simulink model "connections"  (R2020a)
settings: Solver=FixedStepAuto  StartTime=0.0  StopTime=5000  FixedStep=0.1  RelTol=1e-3
values from neighbouring files (symbols this model uses):
  east_drift_limit = 2    [wave_parameters.mat]
  k_down = 1.3    [wave_parameters.mat]
  k_east = 2    [wave_parameters.mat]
  k_north = 2    [wave_parameters.mat]
  k_pitch = 3    [wave_parameters.mat]
  k_roll = 3    [wave_parameters.mat]
  k_yaw = 3    [wave_parameters.mat]
  north_drift_limit = 2    [wave_parameters.mat]
  numberOfBuses = 2    [init.m]
  numberOfGenerators = 4    [init.m]
  peak_frequency = 0.8    [wave_parameters.mat]
  wave_height = 1    [wave_parameters.mat]
  yaw_drift_limit = 0.174532925199    [wave_parameters.mat]
undefined symbols (not defined in the file or in its folder): east, magnitude, north, surge, sway, yaw
libraries: simulink x28, simulink_extras x18
(part 2 of 4)

== system connections/thruster_model/tunnel_thruster_3 ==
  desiredSetPoint : Inport  Unit=N
  desiredAzimuth : Inport  Port=2  Unit=deg
  Abs : Abs
  Add : Sum  Inputs=|+-
  Constant1 : Constant  Value=2
  Constant2 : Constant  Value=3
  Divide : Product
  Gain : Gain  Gain=144000
  Gain1 : Gain  Gain=1/100
  Gain2 : Gain  Gain=925000
  Integrator1 : Integrator
  Power : Math  Operator=pow  SignedPower=on  SaturateOnIntegerOverflow=on
  Power1 : Math  Operator=pow  SignedPower=on  SaturateOnIntegerOverflow=on
  Saturation : Saturate  UpperLimit=100  LowerLimit=-100
  Sign : Signum
  p : Outport  Unit=W  VectorParamsAs1DForOutWhenUnconnected=off  BusOutputAsStruct=on
  thrust : Outport  Port=2  Unit=N  VectorParamsAs1DForOutWhenUnconnected=off
  azimuth : Outport  Port=3  Unit=deg  VectorParamsAs1DForOutWhenUnconnected=off  BusOutputAsStruct=on
  sensorFeedback : Outport  Port=4  Unit=deg  VectorParamsAs1DForOutWhenUnconnected=off  BusOutputAsStruct=on
  wires:
  Abs/1 -> p/1
  Constant1/1 -> Power/2  "q"
  Sign/1 -> Divide/1
  Constant2/1 -> Power1/2  "q"
  Gain2/1 -> Abs/1  "power"
  Gain/1 -> Divide/2  "thrust"
  Power/1 -> Gain/1
  desiredSetPoint/1 -> Saturation/1  "thrustSetPoint"
  Power1/1 -> Gain2/1
  Divide/1 -> thrust/1
  Saturation/1 -> Gain1/1
  Integrator1/1 -> Add/2, Sign/1, sensorFeedback/1, Power1/1, Power/1
  Add/1 -> Integrator1/1
  Gain1/1 -> Add/1
  desiredAzimuth/1 -> azimuth/1

== system connections/vessel_model/VesselDynamics ==
  ExternalForceAndMoments : Inport
  6DOFRotationMatrix : Subsystem
  Add : Sum  Inputs=+--
  Demux : Demux  Outputs=3
  MatrixMultiply : Product  Inputs=/*  Multiplication=Matrix(*)
  MatrixMultiply2 : Product  Inputs=**  Multiplication=Matrix(*)
  Scope : Scope
  Selector : Selector  NumberOfDimensions=2  InputPortWidth=3  IndexOptions=Select all,Index vector (dialog)  Indices=[1 3],1  OutputSizes=1,1
  Selector1 : Selector  InputPortWidth=6  IndexOptions=Index vector (dialog)  Indices=[4 5 6]  OutputSizes=1
  Vessel mass matrix : Constant  Value=diag([3.7e6 5.6e6 5.6e6 2.4e8 1.5e8 7.7e8])
  eta1 : Integrator  InitialCondition=zeros(6,1)  ContinuousStateAttributes='nu'
  linear_damping : Subsystem
  nu1 : Integrator  InitialCondition=zeros(6,1)  ContinuousStateAttributes='eta'
  restoring_forces : Subsystem  mask{a_wp=1548, gm_t=1.5, gm_l=61, rho_w=1025, g=9.81, disp=2000*10}
      mask prompts: a_wp "Water Plane Area"; gm_t "Transverse Metacentric Height"; gm_l "Longitudal Metacentric Height"; rho_w "Density of Water"; g "Gravity"; disp "Displacement"
  eta : Outport  VectorParamsAs1DForOutWhenUnconnected=off
  nu : Outport  Port=2  VectorParamsAs1DForOutWhenUnconnected=off
  wires:
  Demux/2 -> 6DOFRotationMatrix/2(pitch)
  nu1/1 -> Scope/1, MatrixMultiply2/2, linear_damping/1(body_velocity), nu/1  "nu"
  Vessel mass matrix/1 -> MatrixMultiply/1
  Demux/1 -> 6DOFRotationMatrix/1(roll)
  Selector1/1 -> Demux/1
  Demux/3 -> 6DOFRotationMatrix/3(yaw)
  Add/1 -> MatrixMultiply/2
  MatrixMultiply/1 -> Selector/1
  Selector/1 -> nu1/1
  6DOFRotationMatrix/1(6DofRotationMatrix) -> MatrixMultiply2/1
  eta1/1 -> eta/1, restoring_forces/1(ned_position), Selector1/1  "eta"
  ExternalForceAndMoments/1 -> Add/1
  MatrixMultiply2/1 -> eta1/1
  restoring_forces/1(restoring_force) -> Add/3
  linear_damping/1(linear_damping_force) -> Add/2

== system connections/vessel_model/thrust_to_forces ==
  tunnel_thruster_1 : Inport  OutDataTypeStr=Bus: tunnel_thruster
  tunnel_thruster_2 : Inport  Port=2  OutDataTypeStr=Bus: tunnel_thruster
  tunnel_thruster_3 : Inport  Port=3  OutDataTypeStr=Bus: tunnel_thruster
  main_propeller_port : Inport  Port=4  OutDataTypeStr=Bus: azimuth_thruster
  main_propeller_starboard : Inport  Port=5  OutDataTypeStr=Bus: azimuth_thruster
  Bus Selector : BusSelector  OutputSignals=thrust
  Bus Selector1 : BusSelector  OutputSignals=thrust
  Bus Selector2 : BusSelector  OutputSignals=thrust
  Bus Selector3 : BusSelector  OutputSignals=thrust,azimuth
  Bus Selector4 : BusSelector  OutputSignals=thrust,azimuth
  Constant : Constant  Value=90
  Subsystem5 : Subsystem  mask{x=31.25, y=0, z=2.1}
  Subsystem6 : Subsystem  mask{x=24.75, y=0, z=1.9}
  Subsystem7 : Subsystem  mask{x=28.9, y=0, z=1.9}
  Subsystem8 : Subsystem  mask{x=-36.45, y=-4, z=1.415}
  Subsystem9 : Subsystem  mask{x=-36.45, y=4, z=1.415}
  Sum of Elements : Sum  Inputs=+  CollapseMode=Specified dimension  CollapseDim=2
  Vector Concatenate : Concatenate  NumInputs=5  Mode=Multidimensional array  ConcatenateDimension=2
  ForcesAndMomentsvector : Outport  VectorParamsAs1DForOutWhenUnconnected=off
  wires:
  Constant/1 -> Subsystem5/2(alpha), Subsystem6/2(alpha), Subsystem7/2(alpha)
  Sum of Elements/1 -> ForcesAndMomentsvector/1
  Subsystem9/1(Out1) -> Vector Concatenate/5
  Subsystem5/1(Out1) -> Vector Concatenate/1
  Vector Concatenate/1 -> Sum of Elements/1
  Subsystem8/1(Out1) -> Vector Concatenate/4
  Subsystem7/1(Out1) -> Vector Concatenate/2
  Subsystem6/1(Out1) -> Vector Concatenate/3
  tunnel_thruster_1/1 -> Bus Selector/1
  Bus Selector1/1 -> Subsystem7/1(tau)  "<thrust>"
  tunnel_thruster_2/1 -> Bus Selector1/1
  tunnel_thruster_3/1 -> Bus Selector2/1
  Bus Selector2/1 -> Subsystem6/1(tau)  "<thrust>"
  main_propeller_port/1 -> Bus Selector3/1
  Bus Selector3/1 -> Subsystem8/1(tau)  "<thrust>"
  Bus Selector3/2 -> Subsystem8/2(alpha)  "<azimuth>"
  Bus Selector4/2 -> Subsystem9/2(alpha)  "<azimuth>"
  Bus Selector4/1 -> Subsystem9/1(tau)  "<thrust>"
  main_propeller_starboard/1 -> Bus Selector4/1
  Bus Selector/1 -> Subsystem5/1(tau)  "<thrust>"

== system connections/wave_disturbances1/wave_response5 ==
  Hs : Inport
  Band-Limited White Noise : simulink/Sources/Band-Limited White Noise  Cov=0.5  Ts=0.1  seed=[23341]
  C : Gain  Gain=[0 1]  Multiplication=Matrix(K*u)
  Gain : Gain  Gain="[0 1; -peak_frequency^2  -2*0.1017*peak_frequency]"  Multiplication=Matrix(K*u)
  Gain1 : Gain  Gain=[0; 1]  Multiplication=Matrix(K*u)
  Integrator : Integrator  InitialCondition=[0; 0]
  K_w : Subsystem  mask{lambda=0.1017, w0=w0}
      mask prompts: w0 "Peak Frequency"
  MatrixMultiply : Product
  Sum : Sum  Inputs=|++
  Out1 : Outport
  wires:
  Band-Limited White Noise/1 -> Gain1/1
  MatrixMultiply/1 -> Sum/1
  Gain/1 -> Sum/2
  Sum/1 -> Integrator/1
  Gain1/1 -> MatrixMultiply/2
  K_w/1(K_w) -> MatrixMultiply/1
  Hs/1 -> K_w/1(Hs)
  Integrator/1 -> Gain/1, C/1
  C/1 -> Out1/1

== system connections/wave_disturbances1/wave_response_down ==
  Hs : Inport
  Band-Limited White Noise : simulink/Sources/Band-Limited White Noise  Cov=1  Ts=0.1  seed=[23341]
  C : Gain  Gain=[0 1]  Multiplication=Matrix(K*u)
  Gain : Gain  Gain="[0 1; -peak_frequency^2  -2*0.1017*peak_frequency]"  Multiplication=Matrix(K*u)
  Gain1 : Gain  Gain=[0; 1]  Multiplication=Matrix(K*u)
  Integrator : Integrator  InitialCondition=[0; 0]
  K_w : Subsystem  mask{lambda=0.1017, w0=w0}
      mask prompts: w0 "Peak Frequency"
  MatrixMultiply : Product
  Sum : Sum  Inputs=|++
  Out1 : Outport
  wires:
  Integrator/1 -> C/1, Gain/1
  Hs/1 -> K_w/1(Hs)
  K_w/1(K_w) -> MatrixMultiply/1
  Gain1/1 -> MatrixMultiply/2
  Sum/1 -> Integrator/1
  Gain/1 -> Sum/2
  MatrixMultiply/1 -> Sum/1
  Band-Limited White Noise/1 -> Gain1/1
  C/1 -> Out1/1

== system connections/wave_disturbances1/wave_response_east ==
  Hs : Inport
  Band-Limited White Noise : simulink/Sources/Band-Limited White Noise  Cov=1  Ts=0.1  seed=[23341]
  C : Gain  Gain=[0 1]  Multiplication=Matrix(K*u)
  Gain : Gain  Gain="[0 1; -peak_frequency^2  -2*0.1017*peak_frequency]"  Multiplication=Matrix(K*u)
  Gain1 : Gain  Gain=[0; 1]  Multiplication=Matrix(K*u)
  Integrator : Integrator  InitialCondition=[0; 0]
  K_w : Subsystem  mask{lambda=0.1017, w0=w0}
      mask prompts: w0 "Peak Frequency"
  MatrixMultiply : Product
  Sum : Sum  Inputs=|++
  Out1 : Outport
  wires:
  Band-Limited White Noise/1 -> Gain1/1
  MatrixMultiply/1 -> Sum/1
  Gain/1 -> Sum/2
  Sum/1 -> Integrator/1
  Gain1/1 -> MatrixMultiply/2
  K_w/1(K_w) -> MatrixMultiply/1
  Hs/1 -> K_w/1(Hs)
  Integrator/1 -> Gain/1, C/1
  C/1 -> Out1/1

== system connections/wave_disturbances1/wave_response_north ==
  Hs : Inport
  Band-Limited White Noise : simulink/Sources/Band-Limited White Noise  Cov=1  Ts=0.1  seed=[23341]
  C : Gain  Gain=[0 1]  Multiplication=Matrix(K*u)
  Gain : Gain  Gain="[0 1; -peak_frequency^2  -2*0.1017*peak_frequency]"  Multiplication=Matrix(K*u)
  Gain1 : Gain  Gain=[0; 1]  Multiplication=Matrix(K*u)
  Integrator : Integrator  InitialCondition=[0; 0]
  K_w : Subsystem  mask{lambda=0.1017, w0=w0}
      mask prompts: w0 "Peak Frequency"
  MatrixMultiply : Product
  Sum : Sum  Inputs=|++
  Out1 : Outport
  wires:
  Integrator/1 -> C/1, Gain/1
  Hs/1 -> K_w/1(Hs)
  K_w/1(K_w) -> MatrixMultiply/1
  Gain1/1 -> MatrixMultiply/2
  Sum/1 -> Integrator/1
  Gain/1 -> Sum/2
  MatrixMultiply/1 -> Sum/1
  Band-Limited White Noise/1 -> Gain1/1
  C/1 -> Out1/1

== system connections/wave_disturbances1/wave_response_pitch ==
  Hs : Inport
  Band-Limited White Noise : simulink/Sources/Band-Limited White Noise  Cov=1  Ts=0.1  seed=[23341]
  C : Gain  Gain=[0 1]  Multiplication=Matrix(K*u)
  Gain : Gain  Gain="[0 1; -peak_frequency^2  -2*0.1017*peak_frequency]"  Multiplication=Matrix(K*u)
  Gain1 : Gain  Gain=[0; 1]  Multiplication=Matrix(K*u)
  Integrator : Integrator  InitialCondition=[0; 0]
  K_w : Subsystem  mask{lambda=0.1017, w0=w0}
      mask prompts: w0 "Peak Frequency"
  MatrixMultiply : Product
  Sum : Sum  Inputs=|++
  Out1 : Outport
  wires:
  Integrator/1 -> C/1, Gain/1
  Hs/1 -> K_w/1(Hs)
  K_w/1(K_w) -> MatrixMultiply/1
  Gain1/1 -> MatrixMultiply/2
  Sum/1 -> Integrator/1
  Gain/1 -> Sum/2
  MatrixMultiply/1 -> Sum/1
  Band-Limited White Noise/1 -> Gain1/1
  C/1 -> Out1/1

== system connections/wave_disturbances1/wave_response_roll ==
  Hs : Inport
  Band-Limited White Noise : simulink/Sources/Band-Limited White Noise  Cov=1  Ts=0.1  seed=[23341]
  C : Gain  Gain=[0 1]  Multiplication=Matrix(K*u)
  Gain : Gain  Gain="[0 1; -peak_frequency^2  -2*0.1017*peak_frequency]"  Multiplication=Matrix(K*u)
  Gain1 : Gain  Gain=[0; 1]  Multiplication=Matrix(K*u)
  Integrator : Integrator  InitialCondition=[0; 0]
  K_w : Subsystem  mask{lambda=0.1017, w0=w0}
      mask prompts: w0 "Peak Frequency"
  MatrixMultiply : Product
  Sum : Sum  Inputs=|++
  Out1 : Outport
  wires:
  Band-Limited White Noise/1 -> Gain1/1
  MatrixMultiply/1 -> Sum/1
  Gain/1 -> Sum/2
  Sum/1 -> Integrator/1
  Gain1/1 -> MatrixMultiply/2
  K_w/1(K_w) -> MatrixMultiply/1
  Hs/1 -> K_w/1(Hs)
  Integrator/1 -> Gain/1, C/1
  C/1 -> Out1/1

== system connections/winch_controller/referenceModel ==
  In1 : Inport
  Add1 : Sum  Inputs=|+-
  Add2 : Sum  Inputs=|+-
  Gain1 : Gain  Gain=10*10
  Gain2 : Gain  Gain=2*10
  Gain3 : Gain  Gain=10*10
  Integrator : Integrator  LimitOutput=on  UpperSaturationLimit=2  LowerSaturationLimit=-2  ZeroCross=off
  Integrator1 : Integrator  InitialCondition=500  ZeroCross=off
  Saturation1 : Saturate  UpperLimit=200  LowerLimit=-200  ZeroCross=off
  Out1 : Outport  VectorParamsAs1DForOutWhenUnconnected=off
  wires:
  In1/1 -> Gain1/1
  Gain1/1 -> Add2/1
  Add2/1 -> Add1/1
  Saturation1/1 -> Integrator/1
  Integrator1/1 -> Gain3/1, Out1/1
  Gain3/1 -> Add2/2
  Gain2/1 -> Add1/2
  Add1/1 -> Saturation1/1
  Integrator/1 -> Gain2/1, Integrator1/1

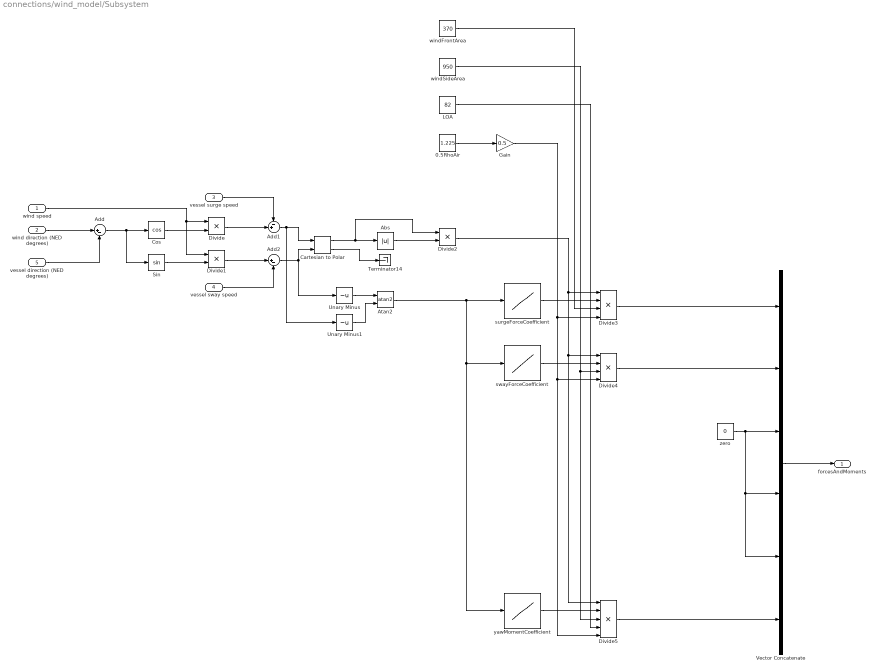
== system connections/wind_model/Subsystem ==
  wind speed : Inport
  wind direction (NED degrees) : Inport  Port=2
  vessel surge speed : Inport  Port=3
  vessel sway speed : Inport  Port=4
  vessel direction (NED degrees) : Inport  Port=5
  0.5RhoAir : Constant  Value=1.225
  Abs : Abs
  Add : Sum  Inputs=|+-
  Add1 : Sum  Inputs=-+|
  Add2 : Sum  Inputs=|+-
  Atan2 : Trigonometry  Operator=atan2
  Cartesian to Polar : simulink_extras/Transformations/Cartesian to Polar
  Cos : Trigonometry  Operator=cos
  Divide : Product
  Divide1 : Product
  Divide2 : Product
  Divide3 : Product  Inputs=4
  Divide4 : Product  Inputs=4
  Divide5 : Product  Inputs=5
  Gain : Gain  Gain=0.5
  LOA : Constant  Value=82
  Sin : Trigonometry
  Terminator14 : Terminator
  Unary Minus : UnaryMinus
  Unary Minus1 : UnaryMinus
  Vector Concatenate : Concatenate  NumInputs=6
  surgeForceCoefficient : Lookup_n-D  NumberOfTableDimensions=1  BreakpointsForDimension1=[0:10:360]  Table=[-0.55 -0.56 -0.50 -0.49 -0.42 -0.34 -0.24 -0.17 -0.11 -0.09 -0.05 0.08 0.39 0.59 0.72 0.80 0.76 0.81 0.80 0.81 0.76 0.80 0.72 0.59 0.39 0.08 -0.05 -0.09 -0.11 -0.17 -0.24 -0.34 -0.42 -0.49 -0.50 -0.56 -0.55]  InternalRulePriority=Speed  RndMeth=Simplest  InputSameDT=on
  swayForceCoefficient : Lookup_n-D  NumberOfTableDimensions=1  BreakpointsForDimension1=[0:10:360]  Table=|  InternalRulePriority=Speed  RndMeth=Simplest  InputSameDT=on
      | [0.0	-0.21	-0.40	-0.60	-0.76	-0.84	-0.95	-0.97	-0.96	-0.92	-0.91	-0.90	-0.86	-0.76	-0.66	-0.51	-0.31	-0.09	0	0.09	0.31	0.51	0.66	0.76	0.86	0.9	0.91	0.92	0.96	0.97	0.95	0.84	0.76	0.6	0.4	0.21	0
      | ]
  windFrontArea : Constant  Value=370
  windSideArea : Constant  Value=950
  yawMomentCoefficient : Lookup_n-D  NumberOfTableDimensions=1  BreakpointsForDimension1=[0:10:360]  Table=|  InternalRulePriority=Speed  RndMeth=Simplest  InputSameDT=on
      | [0.0	-0.060	-0.111	-0.150	-0.160	-0.161	-0.172	-0.162	-0.131	-0.108	-0.071	-0.047	-0.032	-0.008	0.002	0.005	0.007	0.016	0.0	-0.016	-0.007	-0.005	-0.002	0.008	0.032	0.047	0.071	0.108	0.131	0.162	0.172	0.161	0.16	0.15	0.111	0.06	0
      | ]
  zero : Constant  Value=0
  forcesAndMoments : Outport  VectorParamsAs1DForOutWhenUnconnected=off
  wires:
  wind speed/1 -> Divide1/1, Divide/1
  Divide1/1 -> Add2/1
  Gain/1 -> Divide5/5, Divide4/4, Divide3/4
  Add/1 -> Sin/1, Cos/1
  Sin/1 -> Divide1/2
  Divide/1 -> Add1/2
  vessel direction (NED degrees)/1 -> Add/2
  zero/1 -> Vector Concatenate/4, Vector Concatenate/5, Vector Concatenate/3
  wind direction (NED degrees)/1 -> Add/1
  Divide4/1 -> Vector Concatenate/2
  LOA/1 -> Divide5/4
  yawMomentCoefficient/1 -> Divide5/2
  vessel surge speed/1 -> Add1/1
  Divide2/1 -> Divide3/1, Divide4/1, Divide5/1
  Add2/1 -> Unary Minus/1, Cartesian to Polar/2
  windFrontArea/1 -> Divide3/3
  Divide3/1 -> Vector Concatenate/1
  Cartesian to Polar/1 -> Divide2/1, Abs/1
  Divide5/1 -> Vector Concatenate/6
  Add1/1 -> Unary Minus1/1, Cartesian to Polar/1
  Vector Concatenate/1 -> forcesAndMoments/1
  Cartesian to Polar/2 -> Terminator14/1
  surgeForceCoefficient/1 -> Divide3/2
  Atan2/1 -> yawMomentCoefficient/1, swayForceCoefficient/1, surgeForceCoefficient/1
  windSideArea/1 -> Divide5/3, Divide4/3
  Unary Minus/1 -> Atan2/1
  Abs/1 -> Divide2/2
  vessel sway speed/1 -> Add2/2
  Cos/1 -> Divide/2
  0.5RhoAir/1 -> Gain/1
  swayForceCoefficient/1 -> Divide4/2
  Unary Minus1/1 -> Atan2/2

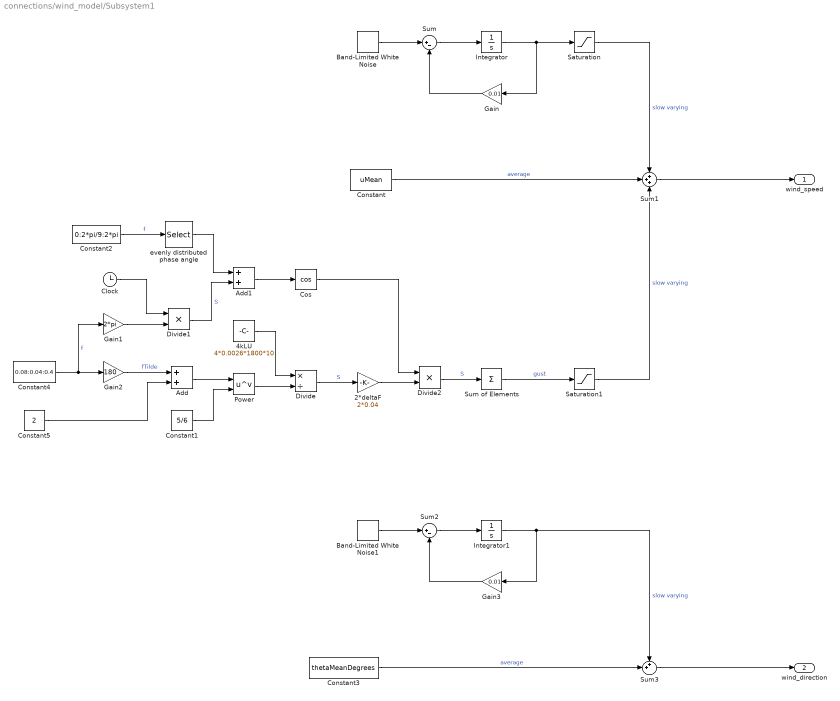
== system connections/wind_model/Subsystem1 ==
  2*deltaF : Gain  Gain=2*0.04
  4kLU : Constant  Value=4*0.0026*1800*10
  Add : Sum
  Add1 : Sum
  Band-Limited White Noise : simulink/Sources/Band-Limited White Noise  Cov=[0.1]  Ts=0.1  seed=[23341]
  Band-Limited White Noise1 : simulink/Sources/Band-Limited White Noise  Cov=[0.1]  Ts=0.1  seed=[23342]
  Clock : Clock
  Constant : Constant  Value=uMean
  Constant1 : Constant  Value=5/6
  Constant2 : Constant  Value=0:2*pi/9:2*pi
  Constant3 : Constant  Value=thetaMeanDegrees
  Constant4 : Constant  Value=0.08:0.04:0.4
  Constant5 : Constant  Value=2
  Cos : Trigonometry  Operator=cos
  Divide : Product  Inputs=*/
  Divide1 : Product
  Divide2 : Product
  Gain : Gain  Gain=0.01
  Gain1 : Gain  Gain=2*pi
  Gain2 : Gain  Gain=180
  Gain3 : Gain  Gain=0.01
  Integrator : Integrator
  Integrator1 : Integrator
  Power : Math  Operator=pow  SignedPower=on  SaturateOnIntegerOverflow=on
  Saturation : Saturate  UpperLimit=uMean/5  LowerLimit=-uMean/5
  Saturation1 : Saturate  UpperLimit=uMean/2  LowerLimit=-uMean/2
  Sum : Sum  Inputs=|+-
  Sum of Elements : Sum  Inputs=+
  Sum1 : Sum  Inputs=+++
  Sum2 : Sum  Inputs=|+-
  Sum3 : Sum  Inputs=++|
  evenly distributed phase angle : Selector  InputPortWidth=10  IndexOptions=Index vector (dialog)  Indices=[1:9]  OutputSizes=1
  wind_speed : Outport  VectorParamsAs1DForOutWhenUnconnected=off
  wind_direction : Outport  Port=2  VectorParamsAs1DForOutWhenUnconnected=off
  wires:
  Band-Limited White Noise1/1 -> Sum2/1
  Constant3/1 -> Sum3/2  "average"
  Gain3/1 -> Sum2/2
  Saturation1/1 -> Sum1/3  "slow varying"
  Gain1/1 -> Divide1/2
  evenly distributed phase angle/1 -> Add1/1
  Sum of Elements/1 -> Saturation1/1  "gust"
  Constant/1 -> Sum1/2  "average"
  Clock/1 -> Divide1/1
  Sum3/1 -> wind_direction/1
  Sum/1 -> Integrator/1
  Sum1/1 -> wind_speed/1
  Integrator1/1 -> Sum3/1, Gain3/1  "slow varying"
  Sum2/1 -> Integrator1/1
  Constant2/1 -> evenly distributed phase angle/1  "f"
  Divide2/1 -> Sum of Elements/1  "S"
  Constant4/1 -> Gain1/1, Gain2/1  "f"
  Add1/1 -> Cos/1
  Integrator/1 -> Gain/1, Saturation/1
  4kLU/1 -> Divide/1
  Divide1/1 -> Add1/2  "S"
  Cos/1 -> Divide2/1
  Gain/1 -> Sum/2
  Divide/1 -> 2*deltaF/1  "S"
  Constant1/1 -> Power/2
  2*deltaF/1 -> Divide2/2
  Constant5/1 -> Add/2
  Add/1 -> Power/1
  Saturation/1 -> Sum1/1  "slow varying"
  Band-Limited White Noise/1 -> Sum/1
  Power/1 -> Divide/2
  Gain2/1 -> Add/1  "fTilde"

== system connections/dp_controller/6DOFRotationMatrix/J1 ==
  yaw : Inport
  pitch : Inport  Port=2
  roll : Inport  Port=3
  Constant1 : Constant
  Constant2 : Constant
  Constant3 : Constant  Value=0
  Constant4 : Constant  Value=0
  Constant5 : Constant
  Constant6 : Constant  Value=0
  Gain : Gain  Gain=-1
  Gain1 : Gain  Gain=-1
  Gain2 : Gain  Gain=-1
  MatrixMultiply : Product  Inputs=3  Multiplication=Matrix(*)
  Reshape : Reshape  OutputDimensionality=Customize  OutputDimensions=[3,3]
  Reshape1 : Reshape  OutputDimensionality=Customize  OutputDimensions=[3,3]
  Reshape2 : Reshape  OutputDimensionality=Customize  OutputDimensions=[3,3]
  Selector : Selector  InputPortWidth=5  IndexOptions=Index vector (dialog)  Indices=[3 4 1 5 3 1 1 1 2]  OutputSizes=1
  Selector3 : Selector  InputPortWidth=5  IndexOptions=Index vector (dialog)  Indices=[3 1 5 1 2 1 4 1 3]  OutputSizes=1
  Selector9 : Selector  InputPortWidth=5  IndexOptions=Index vector (dialog)  Indices=[2 1 1 1 3 4 1 5 3]  OutputSizes=1
  Sin1 : Trigonometry
  Sin2 : Trigonometry
  Sin3 : Trigonometry  Operator=cos
  Sin4 : Trigonometry
  Sin5 : Trigonometry  Operator=cos
  Sin6 : Trigonometry  Operator=cos
  Vector Concatenate2 : Concatenate  NumInputs=5
  Vector Concatenate4 : Concatenate  NumInputs=5
  Vector Concatenate6 : Concatenate  NumInputs=5
  linear rotation matrix : Outport  VectorParamsAs1DForOutWhenUnconnected=off
  wires:
  Sin5/1 -> Vector Concatenate2/3  "cYaw"
  Constant3/1 -> Vector Concatenate2/1
  Constant2/1 -> Vector Concatenate4/2
  Constant4/1 -> Vector Concatenate4/1
  Gain1/1 -> Vector Concatenate4/5
  roll/1 -> Sin6/1, Sin1/1
  Constant1/1 -> Vector Concatenate2/2
  Vector Concatenate4/1 -> Selector3/1
  Vector Concatenate2/1 -> Selector/1
  Reshape2/1 -> MatrixMultiply/1
  Gain/1 -> Vector Concatenate2/5
  Selector9/1 -> Reshape/1
  Vector Concatenate6/1 -> Selector9/1
  Gain2/1 -> Vector Concatenate6/5
  Reshape1/1 -> MatrixMultiply/2
  Selector3/1 -> Reshape1/1
  Sin4/1 -> Gain/1, Vector Concatenate2/4  "sYaw"
  Sin6/1 -> Vector Concatenate6/3  "cYaw"
  Sin2/1 -> Vector Concatenate4/4, Gain1/1  "sYaw"
  Reshape/1 -> MatrixMultiply/3
  yaw/1 -> Sin4/1, Sin5/1
  Selector/1 -> Reshape2/1
  Sin1/1 -> Gain2/1, Vector Concatenate6/4  "sYaw"
  MatrixMultiply/1 -> linear rotation matrix/1
  Constant5/1 -> Vector Concatenate6/2
  Sin3/1 -> Vector Concatenate4/3  "cYaw"
  Constant6/1 -> Vector Concatenate6/1
  pitch/1 -> Sin2/1, Sin3/1

== system connections/dp_controller/6DOFRotationMatrix/J2 ==
  pitch angle : Inport
  roll angle : Inport  Port=2
  Constant : Constant  Value=[1 0 0]
  Gain3 : Gain  Gain=-1
  Reshape3 : Reshape  OutputDimensionality=Customize  OutputDimensions=[3,3]
  Sin10 : Trigonometry  Operator=cos
  Sin7 : Trigonometry
  Sin8 : Trigonometry  Operator=cos
  Sin9 : Trigonometry
  Vector Concatenate : Concatenate  NumInputs=7
  cx/cy : Product  Inputs=/*
  cxty : Product  Inputs=/**
  sx/cy : Product  Inputs=/*
  sxty : Product  Inputs=/**
  angular rotation matrix : Outport  VectorParamsAs1DForOutWhenUnconnected=off
  wires:
  Reshape3/1 -> angular rotation matrix/1
  Gain3/1 -> Vector Concatenate/6
  Constant/1 -> Vector Concatenate/1
  Sin10/1 -> sxty/1, cxty/1, cx/cy/1, sx/cy/1  "cy"
  Vector Concatenate/1 -> Reshape3/1
  cx/cy/1 -> Vector Concatenate/7
  sx/cy/1 -> Vector Concatenate/4
  Sin8/1 -> Vector Concatenate/3, cxty/3, cx/cy/2  "cx"
  cxty/1 -> Vector Concatenate/5
  roll angle/1 -> Sin8/1, Sin7/1
  Sin9/1 -> sxty/2, cxty/2  "sy"
  sxty/1 -> Vector Concatenate/2
  pitch angle/1 -> Sin10/1, Sin9/1
  Sin7/1 -> Gain3/1, sx/cy/2, sxty/3  "sx"

== system connections/power_plant/Subsystem/Bus array to array ==
  powerLoads : Inport  OutDataTypeStr=Bus: swb  Partition=on  PartitionDimension=1  PartitionWidth=1  PartitionOffset=0
  Bus array to array : Subsystem  TreatAsAtomicUnit=on
  For Each : ForEach  DisableCoverage=on
  v : Outport  ConcatenationDimension=1  VectorParamsAs1DForOutWhenUnconnected=off
  w : Outport  Port=2  ConcatenationDimension=1  VectorParamsAs1DForOutWhenUnconnected=off
  theta : Outport  Port=3  ConcatenationDimension=1  VectorParamsAs1DForOutWhenUnconnected=off
  wires:
  powerLoads/1 -> Bus array to array/1(powerLoads)
  Bus array to array/2(w) -> w/1
  Bus array to array/3(theta) -> theta/1
  Bus array to array/1(v) -> v/1

== system connections/power_plant/Subsystem/Bus array to array1 ==
  In1 : Inport  OutDataTypeStr=Bus: TheveninBus  Partition=on  PartitionDimension=1  PartitionWidth=1  PartitionOffset=0
  Bus array to array : Subsystem  TreatAsAtomicUnit=on
  For Each : ForEach  DisableCoverage=on
  E : Outport  ConcatenationDimension=1  VectorParamsAs1DForOutWhenUnconnected=off
  Z : Outport  Port=2  ConcatenationDimension=1  VectorParamsAs1DForOutWhenUnconnected=off
  Sb : Outport  Port=3  ConcatenationDimension=1  VectorParamsAs1DForOutWhenUnconnected=off
  Connected : Outport  Port=4  ConcatenationDimension=1  VectorParamsAs1DForOutWhenUnconnected=off
  omega : Outport  Port=5  ConcatenationDimension=1  VectorParamsAs1DForOutWhenUnconnected=off
  SwitchboardID : Outport  Port=6  ConcatenationDimension=1  VectorParamsAs1DForOutWhenUnconnected=off
  wires:
  Bus array to array/6(SwitchboardID) -> SwitchboardID/1
  Bus array to array/5(omega) -> omega/1
  Bus array to array/4(Connected) -> Connected/1
  Bus array to array/3(Sb) -> Sb/1
  Bus array to array/1(E) -> E/1
  Bus array to array/2(Z) -> Z/1
  In1/1 -> Bus array to array/1(In1)

== system connections/power_plant/Subsystem/Logical selector to find which component is connected to this bus1 ==
  Input : Inport
  Selector : Inport  Port=2
  Relational Operator : RelationalOperator  Operator===  OutDataTypeStr=boolean  RndMeth=Simplest
  Transpose2 : Math  Operator=transpose  SignedPower=on  SaturateOnIntegerOverflow=on
  repmat : Selector  NumberOfDimensions=2  IndexOptions=Index vector (dialog),Index vector (dialog)  Indices=-1,ones(1,numberOfBuses)  OutputSizes=1,1
  repmat1 : Selector  NumberOfDimensions=2  IndexOptions=Index vector (dialog),Index vector (dialog)  Indices=-1,ones(1,numberOfGenerators)  OutputSizes=1,1
  Output : Outport  VectorParamsAs1DForOutWhenUnconnected=off
  wires:
  Transpose2/1 -> Relational Operator/2
  Relational Operator/1 -> Output/1
  repmat1/1 -> Transpose2/1
  repmat/1 -> Relational Operator/1
  Input/1 -> repmat/1
  Selector/1 -> repmat1/1

== system connections/power_plant/Subsystem/Merger ==
  v : Inport  Partition=on  PartitionDimension=1  PartitionWidth=1  PartitionOffset=0
  omega : Inport  Port=2  Partition=on  PartitionDimension=1  PartitionWidth=1  PartitionOffset=0
  theta : Inport  Port=3  Partition=on  PartitionDimension=1  PartitionWidth=1  PartitionOffset=0
  For Each : ForEach  DisableCoverage=on
  For Each Subsystem : Subsystem  TreatAsAtomicUnit=on
  Out1 : Outport  OutDataTypeStr=Bus: swb  ConcatenationDimension=1  VectorParamsAs1DForOutWhenUnconnected=off
  wires:
  For Each Subsystem/1(Out1) -> Out1/1
  v/1 -> For Each Subsystem/1(v)  "voltage"
  omega/1 -> For Each Subsystem/2(omega)  "omega"
  theta/1 -> For Each Subsystem/3(theta)  "thetaElectric"

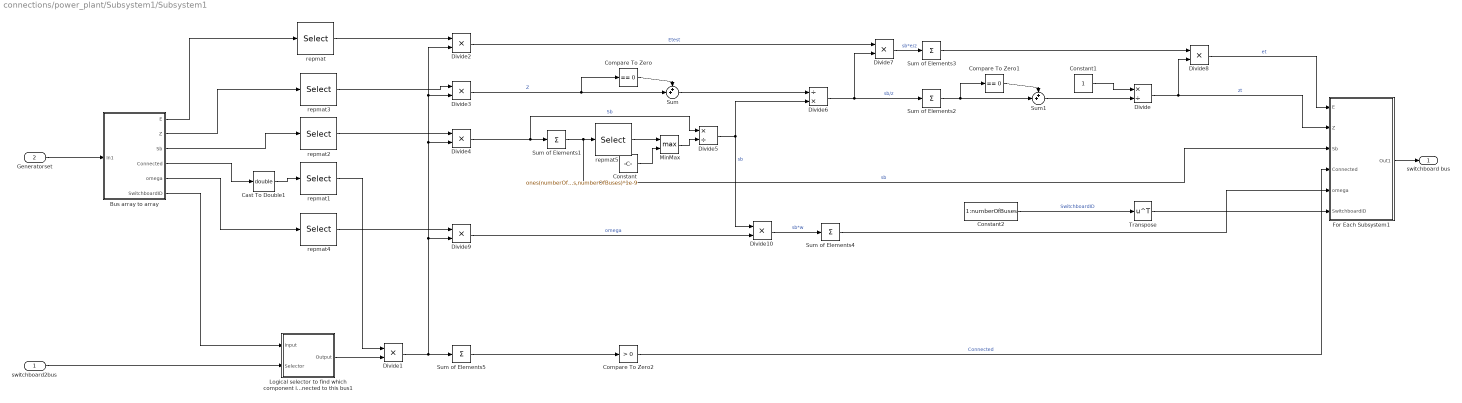
== system connections/power_plant/Subsystem1/Subsystem1 ==
  switchboard2bus : Inport
  Generatorset : Inport  Port=2  OutDataTypeStr=Bus: TheveninBus
  Bus array to array : Subsystem  TreatAsAtomicUnit=on
  Cast To Double1 : DataTypeConversion  OutDataTypeStr=double
  Compare To Zero : simulink/Logic and Bit Operations/Compare To Zero  relop===  OutDataTypeStr=uint8
  Compare To Zero1 : simulink/Logic and Bit Operations/Compare To Zero  relop===  OutDataTypeStr=uint8
  Compare To Zero2 : simulink/Logic and Bit Operations/Compare To Zero  relop=>  OutDataTypeStr=boolean
  Constant : Constant  Value=ones(numberOfGenerators,numberOfBuses)*1e-9
  Constant1 : Constant
  Constant2 : Constant  Value=1:numberOfBuses
  Divide : Product  Inputs=*/
  Divide{1..4,7..10} (8 alike) : Product
  Divide5 : Product  Inputs=*/
  Divide6 : Product  Inputs=/*
  For Each Subsystem1 : Subsystem  TreatAsAtomicUnit=on
  Logical selector to find which component is connected to this bus1 : Subsystem
  MinMax : MinMax  Function=max  Inputs=2
  Sum : Sum  Inputs=++|
  Sum of Elements{1..5} (5 alike) : Sum  Inputs=+  CollapseMode=Specified dimension
  Sum1 : Sum  Inputs=++|
  Transpose : Math  Operator=transpose  SignedPower=on  SaturateOnIntegerOverflow=on
  repmat{,1..4} (5 alike) : Selector  NumberOfDimensions=2  IndexOptions=Index vector (dialog),Index vector (dialog)  Indices=[1 2 3 4],ones(1,numberOfBuses)  OutputSizes=1,1
  repmat5 : Selector  NumberOfDimensions=2  IndexOptions=Index vector (dialog),Index vector (dialog)  Indices=ones(1,numberOfGenerators),-1  OutputSizes=1,1
  switchboard bus : Outport  VectorParamsAs1DForOutWhenUnconnected=off
  wires:
  Cast To Double1/1 -> repmat1/1
  Bus array to array/5(omega) -> repmat4/1
  Generatorset/1 -> Bus array to array/1(In1)
  For Each Subsystem1/1(Out1) -> switchboard bus/1
  Bus array to array/6(SwitchboardID) -> Logical selector to find which component is connected to this bus1/1(Input)
  Bus array to array/3(Sb) -> repmat2/1
  Bus array to array/2(Z) -> repmat3/1
  switchboard2bus/1 -> Logical selector to find which component is connected to this bus1/2(Selector)
  Logical selector to find which component is connected to this bus1/1(Output) -> Divide1/2
  Bus array to array/4(Connected) -> Cast To Double1/1
  repmat2/1 -> Divide4/1
  repmat3/1 -> Divide3/1
  repmat4/1 -> Divide9/1
  repmat1/1 -> Divide1/1
  Divide1/1 -> Divide9/2, Divide2/2, Divide3/2, Divide4/2, Sum of Elements5/1
  Divide4/1 -> Divide5/1, Sum of Elements1/1  "Sb"
  Sum of Elements1/1 -> For Each Subsystem1/3(Sb), repmat5/1  "sb"
  Divide5/1 -> Divide6/2, Divide10/1  "sb"
  repmat5/1 -> MinMax/1
  Constant/1 -> MinMax/2
  MinMax/1 -> Divide5/2
  Divide6/1 -> Divide7/2, Sum of Elements2/1  "sb/z"
  Divide3/1 -> Sum/2, Compare To Zero/1  "Z"
  Compare To Zero/1 -> Sum/1
  Sum/1 -> Divide6/1
  Sum of Elements2/1 -> Sum1/2, Compare To Zero1/1
  Compare To Zero1/1 -> Sum1/1
  Sum1/1 -> Divide/2
  Constant1/1 -> Divide/1
  Divide/1 -> Divide8/2, For Each Subsystem1/2(Z)  "zt"
  Divide7/1 -> Sum of Elements3/1  "sb*e/z"
  Divide2/1 -> Divide7/1  "Etest"
  Sum of Elements3/1 -> Divide8/1
  Divide8/1 -> For Each Subsystem1/1(E)  "et"
  Divide10/1 -> Sum of Elements4/1  "sb*w"
  Divide9/1 -> Divide10/2  "omega"
  Sum of Elements4/1 -> For Each Subsystem1/5(omega)
  Sum of Elements5/1 -> Compare To Zero2/1
  Compare To Zero2/1 -> For Each Subsystem1/4(Connected)  "Connected"
  Constant2/1 -> Transpose/1  "SwitchboardID"
  Transpose/1 -> For Each Subsystem1/6(SwitchboardID)
  Bus array to array/1(E) -> repmat/1
  repmat/1 -> Divide2/1

== system connections/power_plant/Subsystem1/Subsystem2 ==
  loads : Inport
  switchboard2bus : Inport  Port=2
  switchboardBus : Inport  Port=3  LockScale=on
  Bus array to array : Subsystem  TreatAsAtomicUnit=on
  Bus array to array1 : Subsystem  TreatAsAtomicUnit=on
  Compare To Zero : simulink/Logic and Bit Operations/Compare To Zero  relop===  OutDataTypeStr=boolean
  Complex to Magnitude-Angle : ComplexToMagnitudeAngle  Output=Angle
  Logical Operator : Logic  Inputs=1  AllPortsSameDT=off  OutDataTypeStr=boolean
  Logical Operator1 : Logic  Operator=OR  AllPortsSameDT=off  OutDataTypeStr=boolean
  Merger : Subsystem  TreatAsAtomicUnit=on
  Selector : Selector  InputPortWidth=numberOfBuses  IndexOptions=Index vector (port)  Indices=[1 3]  OutputSizes=1
  Terminator : Terminator
  Terminator1 : Terminator
  Terminator2 : Terminator
  busVoltage : Subsystem
  switchboard bus : Outport  OutDataTypeStr=Bus: swb  VectorParamsAs1DForOutWhenUnconnected=off
  isInputValid : Outport  Port=2  VectorParamsAs1DForOutWhenUnconnected=off
  wires:
  busVoltage/1(v) -> Merger/1(v), Complex to Magnitude-Angle/1  "v"
  busVoltage/2(loadAngle) -> Terminator/1
  Selector/1 -> switchboard bus/1
  busVoltage/3(isInputValid) -> Logical Operator1/1
  Logical Operator/1 -> isInputValid/1
  Logical Operator1/1 -> Logical Operator/1
  Complex to Magnitude-Angle/1 -> Merger/3(theta)  "thetaElectric"
  switchboard2bus/1 -> Selector/2
  Bus array to array/6(SwitchboardID) -> Terminator2/1
  Bus array to array/1(E) -> busVoltage/1(ET)
  Bus array to array/2(Z) -> busVoltage/2(ZT)
  Bus array to array/3(Sb) -> busVoltage/3(Sb_bus)
  Bus array to array/4(Connected) -> Compare To Zero/1
  loads/1 -> Bus array to array1/1(SwitchboardBus)
  switchboardBus/1 -> Bus array to array/1(SwitchboardBus)
  Bus array to array1/3(SwitchboardID) -> Terminator1/1
  Merger/1(Out1) -> Selector/1
  Compare To Zero/1 -> Logical Operator1/2
  Bus array to array/5(omega) -> Merger/2(omega)
  Bus array to array1/1(p) -> busVoltage/4(Pbus)
  Bus array to array1/2(q) -> busVoltage/5(Qbus)

== system connections/power_plant/Subsystem1/thrustersToBuses ==
  powerLoads : Inport  OutDataTypeStr=Bus: powerLoadsBus
  s2b : Inport  Port=2
  Bus array to array : Subsystem  TreatAsAtomicUnit=on
  Bus array to array1 : Subsystem  TreatAsAtomicUnit=on
  Divide : Product
  Divide1 : Product
  Logical selector to find which component is connected to this bus : Subsystem
  Sum of Elements : Sum  Inputs=+  CollapseMode=Specified dimension
  Sum of Elements1 : Sum  Inputs=+  CollapseMode=Specified dimension
  Transpose : Math  Operator=transpose  SignedPower=on  SaturateOnIntegerOverflow=on
  repmat : Selector  NumberOfDimensions=2  IndexOptions=Index vector (dialog),Index vector (dialog)  Indices=-1,ones(1,numberOfBuses)  OutputSizes=1,1
  repmat1 : Selector  NumberOfDimensions=2  IndexOptions=Index vector (dialog),Index vector (dialog)  Indices=-1,ones(1,numberOfBuses)  OutputSizes=1,1
  loads : Outport  VectorParamsAs1DForOutWhenUnconnected=off
  wires:
  Divide1/1 -> Sum of Elements1/1
  repmat1/1 -> Divide1/1
  repmat/1 -> Divide/1
  Divide/1 -> Sum of Elements/1
  Sum of Elements1/1 -> Bus array to array1/2(q)  "q"
  Bus array to array1/1(loads) -> loads/1
  powerLoads/1 -> Bus array to array/1(powerLoads)
  s2b/1 -> Transpose/1, Logical selector to find which component is connected to this bus/2(Selector)  "SwitchboardID"
  Bus array to array/3(SwitchboardID) -> Logical selector to find which component is connected to this bus/1(SwitchboardID)
  Logical selector to find which component is connected to this bus/1(Output) -> Divide/2, Divide1/2  "SwitchboardID"
  Bus array to array/1(p) -> repmat/1
  Bus array to array/2(q) -> repmat1/1
  Transpose/1 -> Bus array to array1/3(SwitchboardID)  "SwitchboardID"
  Sum of Elements/1 -> Bus array to array1/1(p)  "p"

== system connections/thruster_model/main_propeller_port/Azimuth Dynamics1 ==
  note: This block calculates the shortest distance for the azimuth to rotate and consider an azimuth speed limit
  Set Point : Inport
  +- 360 if needed : Sum  Inputs=|++
  +- 360 if needed1 : Sum  Inputs=|+-
  Abs : Abs
  Add : Sum  Inputs=|+-
  Constant : Constant  Value=360
  Delay : Delay  DelayLength=1
  Gain1 : Gain  Gain=360
  Gain3 : Gain  Gain=360
  Gain4 : Gain  Gain=-1
  Integrator1 : Integrator  WrappedStateUpperValue=180  WrappedStateLowerValue=-180
  Rem : Math  Operator=rem  SignedPower=on  SaturateOnIntegerOverflow=on
  Sign : Signum
  azimuth speed limit : Saturate  UpperLimit=180  LowerLimit=-180
  change sign : Product
  set-point - currentAngle > 180? : simulink/Logic and Bit Operations/Compare To Constant  relop=>  const=180  OutDataTypeStr=boolean
  set-point - currentAngle > 180?1 : simulink/Logic and Bit Operations/Compare To Constant  relop=>  const=180  OutDataTypeStr=boolean
  currentAngle 0/360 : Outport  VectorParamsAs1DForOutWhenUnconnected=off
  wires:
  +- 360 if needed1/1 -> Delay/1
  set-point - currentAngle > 180?1/1 -> Gain1/1
  Gain1/1 -> +- 360 if needed1/2
  Abs/1 -> set-point - currentAngle > 180?/1
  Rem/1 -> +- 360 if needed1/1, set-point - currentAngle > 180?1/1  "currentAngle"
  set-point - currentAngle > 180?/1 -> Gain3/1
  Delay/1 -> Add/2
  Constant/1 -> Rem/2
  azimuth speed limit/1 -> Integrator1/1
  change sign/1 -> +- 360 if needed/2
  Gain4/1 -> change sign/1
  Gain3/1 -> change sign/2
  Sign/1 -> Gain4/1
  Integrator1/1 -> Rem/1, currentAngle 0/360/1  "azimuthAngle -180/+180"
  Set Point/1 -> Add/1
  Add/1 -> +- 360 if needed/1, Abs/1, Sign/1
  +- 360 if needed/1 -> azimuth speed limit/1

== system connections/thruster_model/main_propeller_port/From degrees to -180//+1 ==
  desiredAzimuth : Inport
  Complex to Magnitude-Angle : ComplexToMagnitudeAngle  Output=Angle
  Degrees to Radians : simulink_extras/Transformations/Degrees to Radians
  Magnitude-Angle to Complex : MagnitudeAngleToComplex  Input=Angle  ConstantPart=1
  Radians to Degrees : simulink_extras/Transformations/Radians to Degrees
  treatedInput : Outport  VectorParamsAs1DForOutWhenUnconnected=off
  wires:
  desiredAzimuth/1 -> Degrees to Radians/1
  Degrees to Radians/1 -> Magnitude-Angle to Complex/1
  Complex to Magnitude-Angle/1 -> Radians to Degrees/1
  Magnitude-Angle to Complex/1 -> Complex to Magnitude-Angle/1
  Radians to Degrees/1 -> treatedInput/1  "treatedInput"

== system connections/thruster_model/main_propeller_port/From degrees to -180//+180 ==
  desiredAzimuth : Inport
  Complex to Magnitude-Angle : ComplexToMagnitudeAngle  Output=Angle
  Degrees to Radians : simulink_extras/Transformations/Degrees to Radians
  Magnitude-Angle to Complex : MagnitudeAngleToComplex  Input=Angle  ConstantPart=1
  Radians to Degrees : simulink_extras/Transformations/Radians to Degrees
  treatedInput : Outport  VectorParamsAs1DForOutWhenUnconnected=off
  wires:
  Radians to Degrees/1 -> treatedInput/1  "treatedInput"
  Magnitude-Angle to Complex/1 -> Complex to Magnitude-Angle/1
  Complex to Magnitude-Angle/1 -> Radians to Degrees/1
  Degrees to Radians/1 -> Magnitude-Angle to Complex/1
  desiredAzimuth/1 -> Degrees to Radians/1

== system connections/thruster_model/main_propeller_starboard/Azimuth Dynamics1 ==
  note: This block calculates the shortest distance for the azimuth to rotate and consider an azimuth speed limit
  Set Point : Inport
  +- 360 if needed : Sum  Inputs=|++
  +- 360 if needed1 : Sum  Inputs=|+-
  Abs : Abs
  Add : Sum  Inputs=|+-
  Constant : Constant  Value=360
  Delay : Delay  DelayLength=1
  Gain1 : Gain  Gain=360
  Gain3 : Gain  Gain=360
  Gain4 : Gain  Gain=-1
  Integrator1 : Integrator  WrappedStateUpperValue=180  WrappedStateLowerValue=-180
  Rem : Math  Operator=rem  SignedPower=on  SaturateOnIntegerOverflow=on
  Sign : Signum
  azimuth speed limit : Saturate  UpperLimit=180  LowerLimit=-180
  change sign : Product
  set-point - currentAngle > 180? : simulink/Logic and Bit Operations/Compare To Constant  relop=>  const=180  OutDataTypeStr=boolean
  set-point - currentAngle > 180?1 : simulink/Logic and Bit Operations/Compare To Constant  relop=>  const=180  OutDataTypeStr=boolean
  currentAngle 0/360 : Outport  VectorParamsAs1DForOutWhenUnconnected=off
  wires:
  +- 360 if needed/1 -> azimuth speed limit/1
  Add/1 -> Sign/1, Abs/1, +- 360 if needed/1
  Set Point/1 -> Add/1
  Integrator1/1 -> currentAngle 0/360/1, Rem/1  "azimuthAngle -180/+180"
  Sign/1 -> Gain4/1
  Gain3/1 -> change sign/2
  Gain4/1 -> change sign/1
  change sign/1 -> +- 360 if needed/2
  azimuth speed limit/1 -> Integrator1/1
  Constant/1 -> Rem/2
  Delay/1 -> Add/2
  set-point - currentAngle > 180?/1 -> Gain3/1
  Rem/1 -> set-point - currentAngle > 180?1/1, +- 360 if needed1/1  "currentAngle"
  Abs/1 -> set-point - currentAngle > 180?/1
  Gain1/1 -> +- 360 if needed1/2
  set-point - currentAngle > 180?1/1 -> Gain1/1
  +- 360 if needed1/1 -> Delay/1

== system connections/thruster_model/main_propeller_starboard/From degrees to -180//+1 ==
  desiredAzimuth : Inport
  Complex to Magnitude-Angle : ComplexToMagnitudeAngle  Output=Angle
  Degrees to Radians : simulink_extras/Transformations/Degrees to Radians
  Magnitude-Angle to Complex : MagnitudeAngleToComplex  Input=Angle  ConstantPart=1
  Radians to Degrees : simulink_extras/Transformations/Radians to Degrees
  treatedInput : Outport  VectorParamsAs1DForOutWhenUnconnected=off
  wires:
  Radians to Degrees/1 -> treatedInput/1  "treatedInput"
  Magnitude-Angle to Complex/1 -> Complex to Magnitude-Angle/1
  Complex to Magnitude-Angle/1 -> Radians to Degrees/1
  Degrees to Radians/1 -> Magnitude-Angle to Complex/1
  desiredAzimuth/1 -> Degrees to Radians/1

== system connections/thruster_model/main_propeller_starboard/From degrees to -180//+180 ==
  desiredAzimuth : Inport
  Complex to Magnitude-Angle : ComplexToMagnitudeAngle  Output=Angle
  Degrees to Radians : simulink_extras/Transformations/Degrees to Radians
  Magnitude-Angle to Complex : MagnitudeAngleToComplex  Input=Angle  ConstantPart=1
  Radians to Degrees : simulink_extras/Transformations/Radians to Degrees
  treatedInput : Outport  VectorParamsAs1DForOutWhenUnconnected=off
  wires:
  desiredAzimuth/1 -> Degrees to Radians/1
  Degrees to Radians/1 -> Magnitude-Angle to Complex/1
  Complex to Magnitude-Angle/1 -> Radians to Degrees/1
  Magnitude-Angle to Complex/1 -> Complex to Magnitude-Angle/1
  Radians to Degrees/1 -> treatedInput/1  "treatedInput"

== system connections/vessel_model/VesselDynamics/6DOFRotationMatrix ==
  roll : Inport
  pitch : Inport  Port=2
  yaw : Inport  Port=3
  J1 : Subsystem
  J2 : Subsystem
  Matrix Concatenate : Concatenate  Mode=Multidimensional array
  Matrix Concatenate1 : Concatenate  Mode=Multidimensional array
  Matrix Concatenate2 : Concatenate  Mode=Multidimensional array  ConcatenateDimension=2
  Zeros : Constant  Value=zeros(3,3)
  6DofRotationMatrix : Outport  VectorParamsAs1DForOutWhenUnconnected=off
  wires:
  pitch/1 -> J1/3(roll), J2/1(pitch angle)
  roll/1 -> J2/2(roll angle), J1/2(pitch)
  Zeros/1 -> Matrix Concatenate/2, Matrix Concatenate1/1
  Matrix Concatenate1/1 -> Matrix Concatenate2/2
  Matrix Concatenate/1 -> Matrix Concatenate2/1
  Matrix Concatenate2/1 -> 6DofRotationMatrix/1
  J2/1(angular rotation matrix) -> Matrix Concatenate1/2
  yaw/1 -> J1/1(yaw)
  J1/1(linear rotation matrix) -> Matrix Concatenate/1

== system connections/vessel_model/VesselDynamics/linear_damping ==
  body_velocity : Inport
  DampingForces : Product  Multiplication=Matrix(*)
  Vessel Damping Matrix : Constant  Value=diag([7.8e3 4.3e4 5.4e6 1.6e9 2.6e9 1.9e7])
  linear_damping_force : Outport  VectorParamsAs1DForOutWhenUnconnected=off
  wires:
  Vessel Damping Matrix/1 -> DampingForces/1
  body_velocity/1 -> DampingForces/2
  DampingForces/1 -> linear_damping_force/1

== system connections/vessel_model/VesselDynamics/restoring_forces ==
  ned_position : Inport  PortDimensions=6
  Constant : Constant  Value=diag([0,0, a_wp, disp*gm_t, disp*gm_l, 0])
  Gain : Gain  Gain=rho_w*g
  MatrixMultiply : Product  Multiplication=Matrix(*)
  restoring_force : Outport  VectorParamsAs1DForOutWhenUnconnected=off
  wires:
  Constant/1 -> Gain/1
  Gain/1 -> MatrixMultiply/1
  ned_position/1 -> MatrixMultiply/2
  MatrixMultiply/1 -> restoring_force/1

== system connections/vessel_model/thrust_to_forces/Subsystem5 ==
  tau : Inport  OutDataTypeStr=double  PortDimensions=1
  alpha : Inport  Port=2  OutDataTypeStr=double  PortDimensions=1
  Add : Sum  Inputs=|+-
  Cos alpha : Trigonometry  Operator=cos
  Degrees to Radians : simulink_extras/Transformations/Degrees to Radians
  Divide{1..5} (5 alike) : Product
  FZ : Constant  Value=0
  Gain : Gain  Gain=-1
  Sin alpha : Trigonometry
  Vector Concatenate1 : Concatenate  NumInputs=6
  x : Constant  Value=x
  y : Constant  Value=y
  z : Constant  Value=z
  Out1 : Outport  OutDataTypeStr=double  PortDimensions=6  VectorParamsAs1DForOutWhenUnconnected=off
  wires:
  Sin alpha/1 -> Divide4/1, Divide1/1, Vector Concatenate1/2
  tau/1 -> Divide2/2
  y/1 -> Divide5/2
  Degrees to Radians/1 -> Sin alpha/1, Cos alpha/1
  Gain/1 -> Vector Concatenate1/4
  z/1 -> Divide1/2, Divide3/1
  Cos alpha/1 -> Divide5/1, Divide3/2, Vector Concatenate1/1
  Divide1/1 -> Gain/1
  Divide5/1 -> Add/2
  Divide2/1 -> Out1/1
  Divide3/1 -> Vector Concatenate1/5
  x/1 -> Divide4/2
  Divide4/1 -> Add/1
  Add/1 -> Vector Concatenate1/6
  FZ/1 -> Vector Concatenate1/3
  Vector Concatenate1/1 -> Divide2/1
  alpha/1 -> Degrees to Radians/1

== system connections/vessel_model/thrust_to_forces/Subsystem6 ==
  tau : Inport  OutDataTypeStr=double  PortDimensions=1
  alpha : Inport  Port=2  OutDataTypeStr=double  PortDimensions=1
  Add : Sum  Inputs=|+-
  Cos alpha : Trigonometry  Operator=cos
  Degrees to Radians : simulink_extras/Transformations/Degrees to Radians
  Divide{1..5} (5 alike) : Product
  FZ : Constant  Value=0
  Gain : Gain  Gain=-1
  Sin alpha : Trigonometry
  Vector Concatenate1 : Concatenate  NumInputs=6
  x : Constant  Value=x
  y : Constant  Value=y
  z : Constant  Value=z
  Out1 : Outport  OutDataTypeStr=double  PortDimensions=6  VectorParamsAs1DForOutWhenUnconnected=off
  wires:
  alpha/1 -> Degrees to Radians/1
  Vector Concatenate1/1 -> Divide2/1
  FZ/1 -> Vector Concatenate1/3
  Add/1 -> Vector Concatenate1/6
  Divide4/1 -> Add/1
  x/1 -> Divide4/2
  Divide3/1 -> Vector Concatenate1/5
  Divide2/1 -> Out1/1
  Divide5/1 -> Add/2
  Divide1/1 -> Gain/1
  Cos alpha/1 -> Vector Concatenate1/1, Divide3/2, Divide5/1
  z/1 -> Divide3/1, Divide1/2
  Gain/1 -> Vector Concatenate1/4
  Degrees to Radians/1 -> Cos alpha/1, Sin alpha/1
  y/1 -> Divide5/2
  tau/1 -> Divide2/2
  Sin alpha/1 -> Vector Concatenate1/2, Divide1/1, Divide4/1

== system connections/vessel_model/thrust_to_forces/Subsystem7 ==
  tau : Inport  OutDataTypeStr=double  PortDimensions=1
  alpha : Inport  Port=2  OutDataTypeStr=double  PortDimensions=1
  Add : Sum  Inputs=|+-
  Cos alpha : Trigonometry  Operator=cos
  Degrees to Radians : simulink_extras/Transformations/Degrees to Radians
  Divide{1..5} (5 alike) : Product
  FZ : Constant  Value=0
  Gain : Gain  Gain=-1
  Sin alpha : Trigonometry
  Vector Concatenate1 : Concatenate  NumInputs=6
  x : Constant  Value=x
  y : Constant  Value=y
  z : Constant  Value=z
  Out1 : Outport  OutDataTypeStr=double  PortDimensions=6  VectorParamsAs1DForOutWhenUnconnected=off
  wires:
  alpha/1 -> Degrees to Radians/1
  Vector Concatenate1/1 -> Divide2/1
  FZ/1 -> Vector Concatenate1/3
  Add/1 -> Vector Concatenate1/6
  Divide4/1 -> Add/1
  x/1 -> Divide4/2
  Divide3/1 -> Vector Concatenate1/5
  Divide2/1 -> Out1/1
  Divide5/1 -> Add/2
  Divide1/1 -> Gain/1
  Cos alpha/1 -> Vector Concatenate1/1, Divide3/2, Divide5/1
  z/1 -> Divide3/1, Divide1/2
  Gain/1 -> Vector Concatenate1/4
  Degrees to Radians/1 -> Cos alpha/1, Sin alpha/1
  y/1 -> Divide5/2
  tau/1 -> Divide2/2
  Sin alpha/1 -> Vector Concatenate1/2, Divide1/1, Divide4/1

== system connections/vessel_model/thrust_to_forces/Subsystem8 ==
  tau : Inport  OutDataTypeStr=double  PortDimensions=1
  alpha : Inport  Port=2  OutDataTypeStr=double  PortDimensions=1
  Add : Sum  Inputs=|+-
  Cos alpha : Trigonometry  Operator=cos
  Degrees to Radians : simulink_extras/Transformations/Degrees to Radians
  Divide{1..5} (5 alike) : Product
  FZ : Constant  Value=0
  Gain : Gain  Gain=-1
  Sin alpha : Trigonometry
  Vector Concatenate1 : Concatenate  NumInputs=6
  x : Constant  Value=x
  y : Constant  Value=y
  z : Constant  Value=z
  Out1 : Outport  OutDataTypeStr=double  PortDimensions=6  VectorParamsAs1DForOutWhenUnconnected=off
  wires:
  Sin alpha/1 -> Divide4/1, Divide1/1, Vector Concatenate1/2
  tau/1 -> Divide2/2
  y/1 -> Divide5/2
  Degrees to Radians/1 -> Sin alpha/1, Cos alpha/1
  Gain/1 -> Vector Concatenate1/4
  z/1 -> Divide1/2, Divide3/1
  Cos alpha/1 -> Divide5/1, Divide3/2, Vector Concatenate1/1
  Divide1/1 -> Gain/1
  Divide5/1 -> Add/2
  Divide2/1 -> Out1/1
  Divide3/1 -> Vector Concatenate1/5
  x/1 -> Divide4/2
  Divide4/1 -> Add/1
  Add/1 -> Vector Concatenate1/6
  FZ/1 -> Vector Concatenate1/3
  Vector Concatenate1/1 -> Divide2/1
  alpha/1 -> Degrees to Radians/1

== system connections/vessel_model/thrust_to_forces/Subsystem9 ==
  tau : Inport  OutDataTypeStr=double  PortDimensions=1
  alpha : Inport  Port=2  OutDataTypeStr=double  PortDimensions=1
  Add : Sum  Inputs=|+-
  Cos alpha : Trigonometry  Operator=cos
  Degrees to Radians : simulink_extras/Transformations/Degrees to Radians
  Divide{1..5} (5 alike) : Product
  FZ : Constant  Value=0
  Gain : Gain  Gain=-1
  Sin alpha : Trigonometry
  Vector Concatenate1 : Concatenate  NumInputs=6
  x : Constant  Value=x
  y : Constant  Value=y
  z : Constant  Value=z
  Out1 : Outport  OutDataTypeStr=double  PortDimensions=6  VectorParamsAs1DForOutWhenUnconnected=off
  wires:
  alpha/1 -> Degrees to Radians/1
  Vector Concatenate1/1 -> Divide2/1
  FZ/1 -> Vector Concatenate1/3
  Add/1 -> Vector Concatenate1/6
  Divide4/1 -> Add/1
  x/1 -> Divide4/2
  Divide3/1 -> Vector Concatenate1/5
  Divide2/1 -> Out1/1
  Divide5/1 -> Add/2
  Divide1/1 -> Gain/1
  Cos alpha/1 -> Vector Concatenate1/1, Divide3/2, Divide5/1
  z/1 -> Divide3/1, Divide1/2
  Gain/1 -> Vector Concatenate1/4
  Degrees to Radians/1 -> Cos alpha/1, Sin alpha/1
  y/1 -> Divide5/2
  tau/1 -> Divide2/2
  Sin alpha/1 -> Vector Concatenate1/2, Divide1/1, Divide4/1

== system connections/wave_disturbances1/wave_response5/K_w ==
  Hs : Inport
  Gain : Gain  Gain=2*lambda*w0
  Sigma : Subsystem
  K_w : Outport
  wires:
  Hs/1 -> Sigma/1(Hs)
  Sigma/1(sigma) -> Gain/1
  Gain/1 -> K_w/1

== system connections/wave_disturbances1/wave_response_down/K_w ==
  Hs : Inport
  Gain : Gain  Gain=2*lambda*w0
  Sigma : Subsystem
  K_w : Outport
  wires:
  Gain/1 -> K_w/1
  Sigma/1(sigma) -> Gain/1
  Hs/1 -> Sigma/1(Hs)

== system connections/wave_disturbances1/wave_response_east/K_w ==
  Hs : Inport
  Gain : Gain  Gain=2*lambda*w0
  Sigma : Subsystem
  K_w : Outport
  wires:
  Hs/1 -> Sigma/1(Hs)
  Sigma/1(sigma) -> Gain/1
  Gain/1 -> K_w/1

== system connections/wave_disturbances1/wave_response_north/K_w ==
  Hs : Inport
  Gain : Gain  Gain=2*lambda*w0
  Sigma : Subsystem
  K_w : Outport
  wires:
  Gain/1 -> K_w/1
  Sigma/1(sigma) -> Gain/1
  Hs/1 -> Sigma/1(Hs)

== system connections/wave_disturbances1/wave_response_pitch/K_w ==
  Hs : Inport
  Gain : Gain  Gain=2*lambda*w0
  Sigma : Subsystem
  K_w : Outport
  wires:
  Gain/1 -> K_w/1
  Sigma/1(sigma) -> Gain/1
  Hs/1 -> Sigma/1(Hs)

== system connections/wave_disturbances1/wave_response_roll/K_w ==
  Hs : Inport
  Gain : Gain  Gain=2*lambda*w0
  Sigma : Subsystem
  K_w : Outport
  wires:
  Hs/1 -> Sigma/1(Hs)
  Sigma/1(sigma) -> Gain/1
  Gain/1 -> K_w/1

== system connections/power_plant/Subsystem/Bus array to array/Bus array to array ==
  powerLoads : Inport  OutDataTypeStr=Bus: swb  Partition=on  PartitionDimension=2  PartitionWidth=1  PartitionOffset=0
  Bus Selector : BusSelector  OutputSignals=voltage,omega,thetaElectric
  For Each : ForEach  DisableCoverage=on
  v : Outport  ConcatenationDimension=2  VectorParamsAs1DForOutWhenUnconnected=off
  w : Outport  Port=2  ConcatenationDimension=2  VectorParamsAs1DForOutWhenUnconnected=off
  theta : Outport  Port=3  ConcatenationDimension=2  VectorParamsAs1DForOutWhenUnconnected=off
  wires:
  powerLoads/1 -> Bus Selector/1
  Bus Selector/2 -> w/1  "<omega>"
  Bus Selector/3 -> theta/1  "<thetaElectric>"
  Bus Selector/1 -> v/1  "<voltage>"
